simulink model "test_switches"  (R2025b)
settings: Solver=VariableStepAuto  StartTime=0.0  StopTime=1  RelTol=1e-3
libraries: fl_lib x28, ee_lib_for_power_systems x21, nesl_utility x7
settings Model: Creator=gdudgeon  LastModifiedBy=gdudgeon
settings RTWCC: GPUComputeCapability=3.5

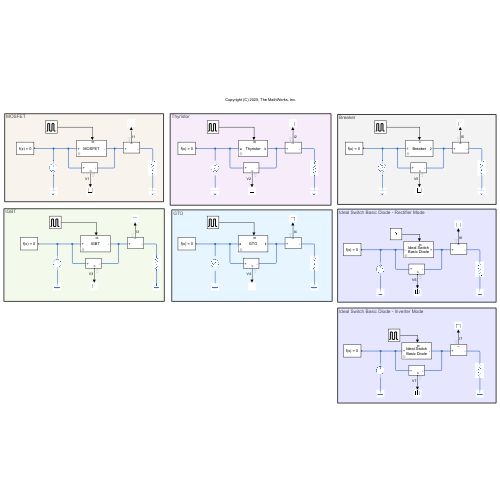
[thumbnail: Simulink's stored preview of the top-level diagram]
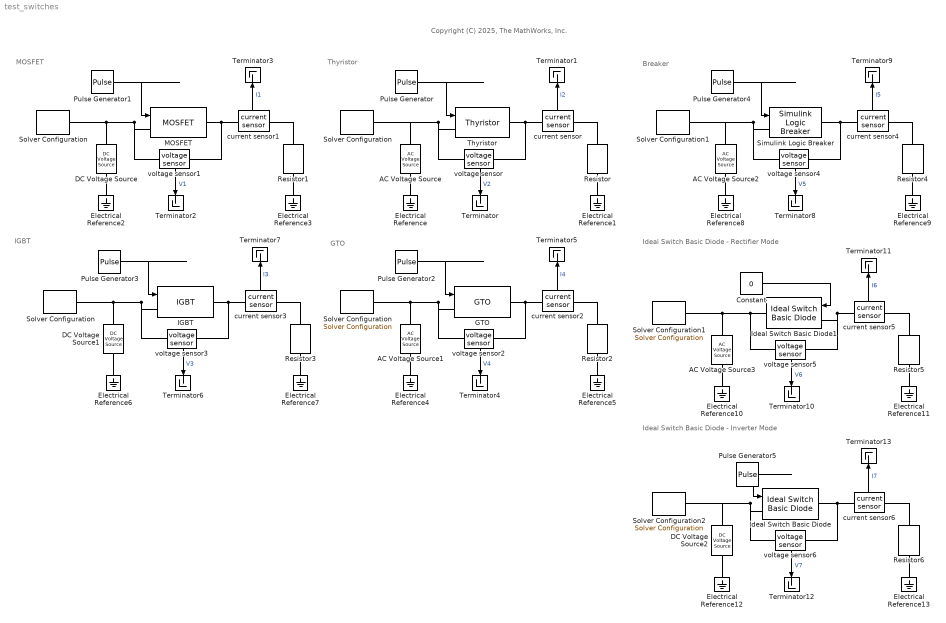
== system test_switches ==
  note: IGBT
  note: MOSFET
  note: Thyristor
  note: Breaker
  note: GTO
  note: Ideal Switch Basic Diode - Rectifier Mode
  note: Copyright (C) 2025, The MathWorks, Inc.
  note: Ideal Switch Basic Diode - Inverter Mode
  " Solver Configuration" : nesl_utility/Solver Configuration  PhysicalDomain=network_engine_domain  SubClassName=solver  LeftPortType=input  RightPortType=generic  Tones=[]  Harmonics=[]  SimulateNoise=off  Profile=off  UseLocalSampling=off  EnableSwitchedLinearOptims=on  FrequencyDomain=off  UseCCode=off  RelTol=0.001  AbsTol=0.001  MinStep=1e-09  ToWorkspace=off  RevertToSquareIcSolve=off  NumHomotopyIterations=100  PhasorMode=off  PhasorModeNumHarmonics=1  ConsistencySolver=NEWTON_XTOL_AFTER_FTOL  IndexReductionMethod=None  DoDC=off  ResidualTolerance=1e-09  ConsistencyTolSource=GLOBAL  ConsistencyAbsTol=0.001  ConsistencyRelTol=0.001  ConsistencyTolFactor=0.001  UseLocalSolver=on  LocalSolverChoice=NE_BACKWARD_EULER_ADVANCER  ResolveIndetEquations=off  FunctionEvalNumThread=1  LocalSolverSampleTime=50e-6  DoFixedCost=on  MaxNonlinIter=2  MaxModeIter=2  ComputeImpulses=off  ImpulseIterations=2  LinearAlgebra=Sparse  LinearAlgebraNumThread=0  EquationFormulation=NE_TIME_EF  DelaysMemoryBudget=1024  AutomaticFiltering=off  FilteringTimeConstant=0.001  PartitionStorageMethod=AS_NEEDED  PartitionMemoryBudget=1024  PartitionMethod=ROBUST  MultibodyUseLocalSolver=off  MultibodyLocalSolverChoice=ODE1  MultibodyLocalSolverSampleTime=0.001
  " Solver Configuration1" : nesl_utility/Solver Configuration  PhysicalDomain=network_engine_domain  SubClassName=solver  LeftPortType=input  RightPortType=generic  Tones=[]  Harmonics=[]  SimulateNoise=off  Profile=off  UseLocalSampling=off  EnableSwitchedLinearOptims=on  FrequencyDomain=off  UseCCode=off  RelTol=0.001  AbsTol=0.001  MinStep=1e-09  ToWorkspace=off  RevertToSquareIcSolve=off  NumHomotopyIterations=100  PhasorMode=off  PhasorModeNumHarmonics=1  ConsistencySolver=NEWTON_XTOL_AFTER_FTOL  IndexReductionMethod=None  DoDC=off  ResidualTolerance=1e-09  ConsistencyTolSource=GLOBAL  ConsistencyAbsTol=0.001  ConsistencyRelTol=0.001  ConsistencyTolFactor=0.001  UseLocalSolver=on  LocalSolverChoice=NE_BACKWARD_EULER_ADVANCER  ResolveIndetEquations=off  FunctionEvalNumThread=1  LocalSolverSampleTime=50e-6  DoFixedCost=on  MaxNonlinIter=2  MaxModeIter=2  ComputeImpulses=off  ImpulseIterations=2  LinearAlgebra=Sparse  LinearAlgebraNumThread=0  EquationFormulation=NE_TIME_EF  DelaysMemoryBudget=1024  AutomaticFiltering=off  FilteringTimeConstant=0.001  PartitionStorageMethod=AS_NEEDED  PartitionMemoryBudget=1024  PartitionMethod=ROBUST  MultibodyUseLocalSolver=off  MultibodyLocalSolverChoice=ODE1  MultibodyLocalSolverSampleTime=0.001
  " Solver Configuration2" : nesl_utility/Solver Configuration  PhysicalDomain=network_engine_domain  SubClassName=solver  LeftPortType=input  RightPortType=generic  Tones=[]  Harmonics=[]  SimulateNoise=off  Profile=off  UseLocalSampling=off  EnableSwitchedLinearOptims=on  FrequencyDomain=off  UseCCode=off  RelTol=0.001  AbsTol=0.001  MinStep=1e-09  ToWorkspace=off  RevertToSquareIcSolve=off  NumHomotopyIterations=100  PhasorMode=off  PhasorModeNumHarmonics=1  ConsistencySolver=NEWTON_XTOL_AFTER_FTOL  IndexReductionMethod=None  DoDC=off  ResidualTolerance=1e-09  ConsistencyTolSource=GLOBAL  ConsistencyAbsTol=0.001  ConsistencyRelTol=0.001  ConsistencyTolFactor=0.001  UseLocalSolver=on  LocalSolverChoice=NE_BACKWARD_EULER_ADVANCER  ResolveIndetEquations=off  FunctionEvalNumThread=1  LocalSolverSampleTime=50e-6  DoFixedCost=on  MaxNonlinIter=2  MaxModeIter=2  ComputeImpulses=off  ImpulseIterations=2  LinearAlgebra=Sparse  LinearAlgebraNumThread=0  EquationFormulation=NE_TIME_EF  DelaysMemoryBudget=1024  AutomaticFiltering=off  FilteringTimeConstant=0.001  PartitionStorageMethod=AS_NEEDED  PartitionMemoryBudget=1024  PartitionMethod=ROBUST  MultibodyUseLocalSolver=off  MultibodyLocalSolverChoice=ODE1  MultibodyLocalSolverSampleTime=0.001
  AC Voltage Source{,1..3} (4 alike) : fl_lib/Electrical/Electrical Sources/AC Voltage Source  amp=1 V  shift=0 deg  frequency=10 Hz
  Constant : Constant  Value=0
  DC Voltage Source : fl_lib/Electrical/Electrical Sources/DC Voltage Source  v0=1 V
  DC Voltage Source1 : fl_lib/Electrical/Electrical Sources/DC Voltage Source  v0=1 V
  DC Voltage Source2 : fl_lib/Electrical/Electrical Sources/DC Voltage Source  v0=1 V
  Electrical Reference{,1..13} (14 alike) : fl_lib/Electrical/Electrical Elements/Electrical Reference
  GTO : ee_lib_for_power_systems/Power Converters/GTO  Ron=1e-5  Goff=1e-5  Vf=0.6  run_time=off
      settings: SourceProductName=Support Library for Power Systems
  IGBT : ee_lib_for_power_systems/Power Converters/IGBT  Vf=0.6  Ron=1e-3  Goff=1e-5  run_time=off
      settings: SourceProductName=Support Library for Power Systems
  Ideal Switch Basic Diode : ee_lib_for_power_systems/Power Converters/Ideal Switch Basic Diode  Ron=1e-3  Goff=1e-5  run_time=off
      settings: SourceProductName=Support Library for Power Systems
  Ideal Switch Basic Diode1 : ee_lib_for_power_systems/Power Converters/Ideal Switch Basic Diode  Ron=1e-3  Goff=1e-5  run_time=off
      settings: SourceProductName=Support Library for Power Systems
  MOSFET : ee_lib_for_power_systems/Power Converters/MOSFET  Ron=1e-3  Goff=1e-5  run_time=off
      settings: SourceProductName=Support Library for Power Systems
  Pulse Generator{,1..3,5} (5 alike) : DiscretePulseGenerator  PulseType=Time based  Period=0.1  PulseWidth=50
  Pulse Generator4 : DiscretePulseGenerator  PulseType=Time based  Period=0.1  PulseWidth=50  PhaseDelay=0.1/4
  Resistor{,1..6} (7 alike) : fl_lib/Electrical/Electrical Elements/Resistor  R=1 Ohm  i_specify=off  i_priority=None  i=0 A  i_nominal_specify=off  i_nominal_value=1  i_nominal_unit=A  v_specify=off  v_priority=None  v=0 V  v_nominal_specify=off  v_nominal_value=1  v_nominal_unit=V
  Simulink Logic Breaker : ee_lib_for_power_systems/Network Components/Simulink Logic Breaker  initB=1  Ron=1e-6  Goff=1e-6  Ts=5e-5
      settings: SourceProductName=Support Library for Power Systems
  Solver Configuration : nesl_utility/Solver Configuration  PhysicalDomain=network_engine_domain  SubClassName=solver  LeftPortType=input  RightPortType=generic  Tones=[]  Harmonics=[]  SimulateNoise=off  Profile=off  UseLocalSampling=off  EnableSwitchedLinearOptims=on  FrequencyDomain=off  UseCCode=off  RelTol=0.001  AbsTol=0.001  MinStep=1e-09  ToWorkspace=off  RevertToSquareIcSolve=off  NumHomotopyIterations=100  PhasorMode=off  PhasorModeNumHarmonics=1  ConsistencySolver=NEWTON_XTOL_AFTER_FTOL  IndexReductionMethod=None  DoDC=off  ResidualTolerance=1e-09  ConsistencyTolSource=GLOBAL  ConsistencyAbsTol=0.001  ConsistencyRelTol=0.001  ConsistencyTolFactor=0.001  UseLocalSolver=on  LocalSolverChoice=NE_BACKWARD_EULER_ADVANCER  ResolveIndetEquations=off  FunctionEvalNumThread=1  LocalSolverSampleTime=50e-6  DoFixedCost=on  MaxNonlinIter=2  MaxModeIter=2  ComputeImpulses=off  ImpulseIterations=2  LinearAlgebra=Sparse  LinearAlgebraNumThread=0  EquationFormulation=NE_TIME_EF  DelaysMemoryBudget=1024  AutomaticFiltering=off  FilteringTimeConstant=0.001  PartitionStorageMethod=AS_NEEDED  PartitionMemoryBudget=1024  PartitionMethod=ROBUST  MultibodyUseLocalSolver=off  MultibodyLocalSolverChoice=ODE1  MultibodyLocalSolverSampleTime=0.001
  "Solver Configuration " : nesl_utility/Solver Configuration  PhysicalDomain=network_engine_domain  SubClassName=solver  LeftPortType=input  RightPortType=generic  Tones=[]  Harmonics=[]  SimulateNoise=off  Profile=off  UseLocalSampling=off  EnableSwitchedLinearOptims=on  FrequencyDomain=off  UseCCode=off  RelTol=0.001  AbsTol=0.001  MinStep=1e-09  ToWorkspace=off  RevertToSquareIcSolve=off  NumHomotopyIterations=100  PhasorMode=off  PhasorModeNumHarmonics=1  ConsistencySolver=NEWTON_XTOL_AFTER_FTOL  IndexReductionMethod=None  DoDC=off  ResidualTolerance=1e-09  ConsistencyTolSource=GLOBAL  ConsistencyAbsTol=0.001  ConsistencyRelTol=0.001  ConsistencyTolFactor=0.001  UseLocalSolver=on  LocalSolverChoice=NE_BACKWARD_EULER_ADVANCER  ResolveIndetEquations=off  FunctionEvalNumThread=1  LocalSolverSampleTime=50e-6  DoFixedCost=on  MaxNonlinIter=2  MaxModeIter=2  ComputeImpulses=off  ImpulseIterations=2  LinearAlgebra=Sparse  LinearAlgebraNumThread=0  EquationFormulation=NE_TIME_EF  DelaysMemoryBudget=1024  AutomaticFiltering=off  FilteringTimeConstant=0.001  PartitionStorageMethod=AS_NEEDED  PartitionMemoryBudget=1024  PartitionMethod=ROBUST  MultibodyUseLocalSolver=off  MultibodyLocalSolverChoice=ODE1  MultibodyLocalSolverSampleTime=0.001
  "Solver Configuration  " : nesl_utility/Solver Configuration  PhysicalDomain=network_engine_domain  SubClassName=solver  LeftPortType=input  RightPortType=generic  Tones=[]  Harmonics=[]  SimulateNoise=off  Profile=off  UseLocalSampling=off  EnableSwitchedLinearOptims=on  FrequencyDomain=off  UseCCode=off  RelTol=0.001  AbsTol=0.001  MinStep=1e-09  ToWorkspace=off  RevertToSquareIcSolve=off  NumHomotopyIterations=100  PhasorMode=off  PhasorModeNumHarmonics=1  ConsistencySolver=NEWTON_XTOL_AFTER_FTOL  IndexReductionMethod=None  DoDC=off  ResidualTolerance=1e-09  ConsistencyTolSource=GLOBAL  ConsistencyAbsTol=0.001  ConsistencyRelTol=0.001  ConsistencyTolFactor=0.001  UseLocalSolver=on  LocalSolverChoice=NE_BACKWARD_EULER_ADVANCER  ResolveIndetEquations=off  FunctionEvalNumThread=1  LocalSolverSampleTime=50e-6  DoFixedCost=on  MaxNonlinIter=2  MaxModeIter=2  ComputeImpulses=off  ImpulseIterations=2  LinearAlgebra=Sparse  LinearAlgebraNumThread=0  EquationFormulation=NE_TIME_EF  DelaysMemoryBudget=1024  AutomaticFiltering=off  FilteringTimeConstant=0.001  PartitionStorageMethod=AS_NEEDED  PartitionMemoryBudget=1024  PartitionMethod=ROBUST  MultibodyUseLocalSolver=off  MultibodyLocalSolverChoice=ODE1  MultibodyLocalSolverSampleTime=0.001
  Solver Configuration1 : nesl_utility/Solver Configuration  PhysicalDomain=network_engine_domain  SubClassName=solver  LeftPortType=input  RightPortType=generic  Tones=[]  Harmonics=[]  SimulateNoise=off  Profile=off  UseLocalSampling=off  EnableSwitchedLinearOptims=on  FrequencyDomain=off  UseCCode=off  RelTol=0.001  AbsTol=0.001  MinStep=1e-09  ToWorkspace=off  RevertToSquareIcSolve=off  NumHomotopyIterations=100  PhasorMode=off  PhasorModeNumHarmonics=1  ConsistencySolver=NEWTON_XTOL_AFTER_FTOL  IndexReductionMethod=None  DoDC=off  ResidualTolerance=1e-09  ConsistencyTolSource=GLOBAL  ConsistencyAbsTol=0.001  ConsistencyRelTol=0.001  ConsistencyTolFactor=0.001  UseLocalSolver=on  LocalSolverChoice=NE_BACKWARD_EULER_ADVANCER  ResolveIndetEquations=off  FunctionEvalNumThread=1  LocalSolverSampleTime=50e-6  DoFixedCost=on  MaxNonlinIter=2  MaxModeIter=2  ComputeImpulses=off  ImpulseIterations=2  LinearAlgebra=Sparse  LinearAlgebraNumThread=0  EquationFormulation=NE_TIME_EF  DelaysMemoryBudget=1024  AutomaticFiltering=off  FilteringTimeConstant=0.001  PartitionStorageMethod=AS_NEEDED  PartitionMemoryBudget=1024  PartitionMethod=ROBUST  MultibodyUseLocalSolver=off  MultibodyLocalSolverChoice=ODE1  MultibodyLocalSolverSampleTime=0.001
  Terminator{,1..13} (14 alike) : Terminator
  Thyristor : ee_lib_for_power_systems/Power Converters/Thyristor  Ron=1e-5  Goff=1e-5  Vf=0.6  run_time=off
      settings: SourceProductName=Support Library for Power Systems
  current sensor{,1..6} (7 alike) : ee_lib_for_power_systems/Sense and Measure/current sensor  SystemSampleTime=-1  VariantActivationTime=update diagram  EmptyChoice=off  PassThrough=off  PassThroughVariantControl=(default)  EmptyChoiceVariantControl=(default)  AllowFlexibleInterface=on  Latency=0  AutoFrameSizeCalculation=off
      settings: SourceProductName=Support Library for Power Systems  PortSchema="{\"entries\":[{\"content\":{\"sides\":[{\"content\":{\"connectorIds\":[\"LConn1\"]},\"type\":\"ConnectorPlacement.EquallySpacedRectSide\",\"uuid\":\"799648ba-196f-427a-9565-f64fffdae700\"},{\"content\":{\"connectorIds\":[\"RConn1\"],\"side\":\"RIGHT\"},\"type\":\"ConnectorPlacement.EquallySpacedRectSide\",\"uuid\":\"662de5d5-c2ef-406c-9235-94a35f9d89fb\"},{\"content\":{\"connectorIds\":[\"Out1\"],\"side\":\"TOP\"},\"type\":\"ConnectorPlacement.EquallySpacedRectSide\",\"uuid\":\"67dc8fec-98bd-426f-bbe6-5723f2587b12\"}]},\"type\":\"ConnectorPlacement.EquallySpacedConnector\",\"uuid\":\"3e33dbb3-529a-4788-9727-18d62c402281\"}],\"packageUris\":[\"http://schema.mathworks.com/mf0/Connector/R2020b\"],\"version\":\"1.0\"}"
  voltage sensor{,1..6} (7 alike) : ee_lib_for_power_systems/Sense and Measure/voltage sensor  SystemSampleTime=-1  VariantActivationTime=update diagram  EmptyChoice=off  PassThrough=off  PassThroughVariantControl=(default)  EmptyChoiceVariantControl=(default)  AllowFlexibleInterface=on  Latency=0  AutoFrameSizeCalculation=off
      settings: SourceProductName=Support Library for Power Systems  PortSchema="{\"entries\":[{\"content\":{\"sides\":[{\"content\":{},\"type\":\"ConnectorPlacement.EquallySpacedRectSide\",\"uuid\":\"799648ba-196f-427a-9565-f64fffdae700\"},{\"content\":{\"connectorIds\":[\"Out1\"],\"side\":\"RIGHT\"},\"type\":\"ConnectorPlacement.EquallySpacedRectSide\",\"uuid\":\"662de5d5-c2ef-406c-9235-94a35f9d89fb\"},{\"content\":{\"connectorIds\":[\"LConn1\"],\"side\":\"TOP\"},\"type\":\"ConnectorPlacement.EquallySpacedRectSide\",\"uuid\":\"67dc8fec-98bd-426f-bbe6-5723f2587b12\"},{\"content\":{\"connectorIds\":[\"RConn1\"],\"side\":\"BOTTOM\"},\"type\":\"ConnectorPlacement.EquallySpacedRectSide\",\"uuid\":\"7e3d7354-1ab6-44d8-9b44-c988118d052c\"}]},\"type\":\"ConnectorPlacement.EquallySpacedConnector\",\"uuid\":\"3e33dbb3-529a-4788-9727-18d62c402281\"}],\"packageUris\":[\"http://schema.mathworks.com/mf0/Connector/R2020b\"],\"version\":\"1.0\"}"
  wires:
  voltage sensor/1 -> Terminator/1  "V2"
  current sensor/1 -> Terminator1/1  "I2"
  Pulse Generator/1 -> Thyristor/1
  Pulse Generator1/1 -> MOSFET/1
  current sensor1/1 -> Terminator3/1  "I1"
  voltage sensor1/1 -> Terminator2/1  "V1"
  voltage sensor3/1 -> Terminator6/1  "V3"
  current sensor3/1 -> Terminator7/1  "I3"
  Pulse Generator3/1 -> IGBT/1
  Pulse Generator2/1 -> GTO/1
  current sensor2/1 -> Terminator5/1  "I4"
  voltage sensor2/1 -> Terminator4/1  "V4"
  Pulse Generator4/1 -> Simulink Logic Breaker/1
  current sensor4/1 -> Terminator9/1  "I5"
  voltage sensor4/1 -> Terminator8/1  "V5"
  voltage sensor5/1 -> Terminator10/1  "V6"
  current sensor5/1 -> Terminator11/1  "I6"
  Constant/1 -> Ideal Switch Basic Diode1/1
  Pulse Generator5/1 -> Ideal Switch Basic Diode/1
  current sensor6/1 -> Terminator13/1  "I7"
  voltage sensor6/1 -> Terminator12/1  "V7"
  connections:
  voltage sensor/LConn1 -- Thyristor/LConn1 -- AC Voltage Source/LConn1 -- Solver Configuration/RConn1
  AC Voltage Source/RConn1 -- Electrical Reference/LConn1
  current sensor/LConn1 -- Thyristor/RConn1 -- voltage sensor/RConn1
  Resistor/LConn1 -- current sensor/RConn1
  Electrical Reference1/LConn1 -- Resistor/RConn1
  "Solver Configuration "/RConn1 -- DC Voltage Source/LConn1 -- MOSFET/LConn1 -- voltage sensor1/LConn1
  voltage sensor1/RConn1 -- MOSFET/RConn1 -- current sensor1/LConn1
  Electrical Reference3/LConn1 -- Resistor1/RConn1
  DC Voltage Source/RConn1 -- Electrical Reference2/LConn1
  Resistor1/LConn1 -- current sensor1/RConn1
  AC Voltage Source1/LConn1 -- " Solver Configuration"/RConn1 -- GTO/LConn1 -- voltage sensor2/LConn1
  voltage sensor2/RConn1 -- GTO/RConn1 -- current sensor2/LConn1
  DC Voltage Source1/LConn1 -- IGBT/LConn1 -- voltage sensor3/LConn1 -- "Solver Configuration  "/RConn1
  current sensor3/LConn1 -- IGBT/RConn1 -- voltage sensor3/RConn1
  Resistor3/LConn1 -- current sensor3/RConn1
  DC Voltage Source1/RConn1 -- Electrical Reference6/LConn1
  Electrical Reference7/LConn1 -- Resistor3/RConn1
  Electrical Reference5/LConn1 -- Resistor2/RConn1
  AC Voltage Source1/RConn1 -- Electrical Reference4/LConn1
  Resistor2/LConn1 -- current sensor2/RConn1
  voltage sensor4/LConn1 -- Simulink Logic Breaker/LConn1 -- Solver Configuration1/RConn1 -- AC Voltage Source2/LConn1
  current sensor4/LConn1 -- Simulink Logic Breaker/RConn1 -- voltage sensor4/RConn1
  Resistor4/LConn1 -- current sensor4/RConn1
  AC Voltage Source2/RConn1 -- Electrical Reference8/LConn1
  Electrical Reference9/LConn1 -- Resistor4/RConn1
  AC Voltage Source3/LConn1 -- Ideal Switch Basic Diode1/RConn1 -- voltage sensor5/LConn1 -- " Solver Configuration1"/RConn1
  voltage sensor5/RConn1 -- Ideal Switch Basic Diode1/LConn1 -- current sensor5/LConn1
  Resistor5/LConn1 -- current sensor5/RConn1
  AC Voltage Source3/RConn1 -- Electrical Reference10/LConn1
  Electrical Reference11/LConn1 -- Resistor5/RConn1
  DC Voltage Source2/LConn1 -- " Solver Configuration2"/RConn1 -- voltage sensor6/LConn1 -- Ideal Switch Basic Diode/LConn1
  voltage sensor6/RConn1 -- Ideal Switch Basic Diode/RConn1 -- current sensor6/LConn1
  Electrical Reference13/LConn1 -- Resistor6/RConn1
  Resistor6/LConn1 -- current sensor6/RConn1
  DC Voltage Source2/RConn1 -- Electrical Reference12/LConn1
